simulink model "UR5"  (R2021a)
settings: Solver=ode45  StartTime=0.0  StopTime=duration  MaxStep=0.0001  RelTol=1e-3
values from neighbouring files (symbols this model uses):
  bound = 1e-6    (= 1e-06)    [parameter_setting.m]
  degree = 0.5    [parameter_setting.m]
  N = 2    [ICL_offline.m]
  rp = [-0.1 0 0.1]    [parameter_setting.m]
undefined symbols (not defined in the file or in its folder): DiscIntNeverNeededParam, Levenberg, Marquardt, sigbuilder_block, X, Y, Z
libraries: sm_lib x166, nesl_utility x41, robotmaniplib x2, SignalEditorBlockLib x2
(part 5 of 5)

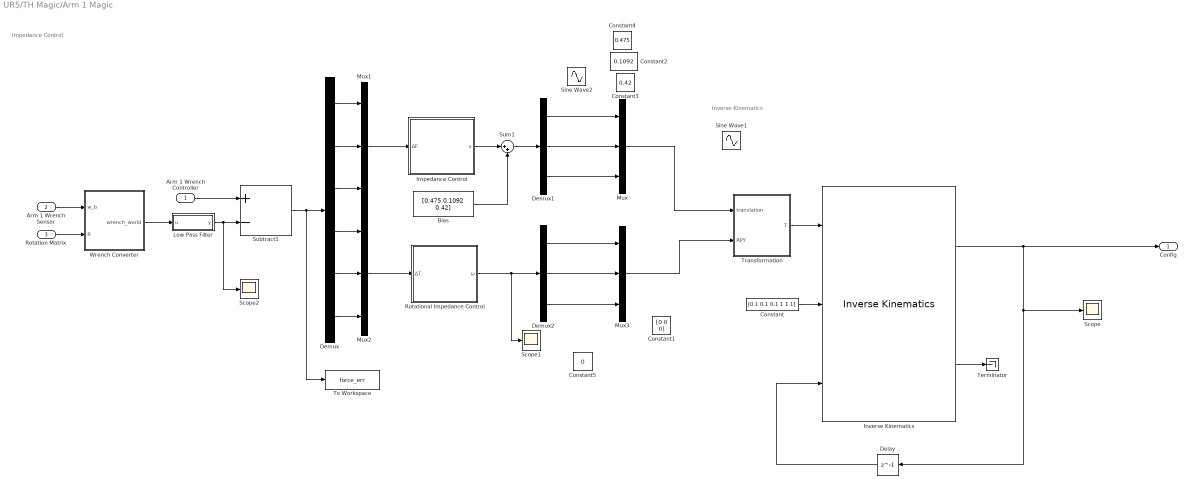
== system UR5/TH Magic/Arm 1 Magic ==
  note: Impedance Control
  note: Inverse Kinematics
  Arm 1 Wrench Controller : Inport
  Arm 1 Wrench Sensor : Inport  Port=2
  Rotation Matrix : Inport  Port=3
  Bias : Constant  Value=[0.475 0.1092 0.42]
  Constant : Constant  Value=[0.1 0.1 0.1 1 1 1]
  Constant1 : Constant  Value=[0 0 0]
  Constant2 : Constant  Value=0.1092
  Constant3 : Constant  Value=0.42
  Constant4 : Constant  Value=0.475
  Constant5 : Constant  Value=0
  Delay : Delay  DelayLength=1
  Demux : Demux  Outputs=6
  Demux1 : Demux  Outputs=3
  Demux2 : Demux  Outputs=3
  Impedance Control : Subsystem
  Inverse Kinematics : robotmaniplib/Inverse Kinematics  RigidBodyTree=robot  EndEffector=ee_link  ShowInfo=on  SolverName=Levenberg-Marquardt  EnforceJointLimits=on  MaxIterations=1500  MaxTime=10  GradientTolerance=1e-7  SolutionTolerance=1e-6  StepTolerance=1e-14  ErrorChangeTolerance=1e-12  UseErrorDamping=on  DampingBias=0.0025  SimulateUsing=Interpreted execution
  Low Pass Filter : MATLAB Function  TreatAsAtomicUnit=on
  Mux{,1..3} (4 alike) : Mux  Inputs=3
  Rotational Impedance Control : Subsystem
  Scope : Scope
  Scope1 : Scope
  Scope2 : Scope
  Sine Wave1 : Sin  Amplitude=0.2  Bias=0.475  Frequency=1.6  SampleTime=0
  Sine Wave2 : Sin  Amplitude=-0.2  Bias=0.475  Frequency=1.6  SampleTime=0
  Subtract1 : Sum  Inputs=+-
  Sum1 : Sum  Inputs=|++
  Terminator : Terminator
  To Workspace : ToWorkspace  VariableName=force_err  SaveFormat=Timeseries  SampleTime=-1
  Transformation : MATLAB Function  TreatAsAtomicUnit=on
  Wrench Converter : MATLAB Function  TreatAsAtomicUnit=on
  Config : Outport
  wires:
  Demux/3 -> Mux1/3
  Mux/1 -> Transformation/1(translation)
  Inverse Kinematics/1 -> Config/1, Delay/1, Scope/1
  Transformation/1(T) -> Inverse Kinematics/1
  Demux/6 -> Mux2/3
  Demux/5 -> Mux2/2
  Bias/1 -> Sum1/2
  Inverse Kinematics/2 -> Terminator/1
  Constant/1 -> Inverse Kinematics/2
  Demux/2 -> Mux1/2
  Delay/1 -> Inverse Kinematics/3
  Demux/1 -> Mux1/1
  Mux2/1 -> Rotational Impedance Control/1(ΔT)
  Rotational Impedance Control/1(ω) -> Scope1/1, Demux2/1
  Demux/4 -> Mux2/1
  Mux1/1 -> Impedance Control/1(ΔF)
  Demux1/3 -> Mux/3
  Subtract1/1 -> To Workspace/1, Demux/1
  Arm 1 Wrench Controller/1 -> Subtract1/1
  Arm 1 Wrench Sensor/1 -> Wrench Converter/1(w_b)
  Rotation Matrix/1 -> Wrench Converter/2(R)
  Sum1/1 -> Demux1/1
  Demux1/2 -> Mux/2
  Demux2/2 -> Mux3/2
  Demux2/1 -> Mux3/1
  Demux2/3 -> Mux3/3
  Demux1/1 -> Mux/1
  Impedance Control/1(x) -> Sum1/1
  Mux3/1 -> Transformation/2(RPY)
  Wrench Converter/1(wrench_world) -> Low Pass Filter/1(u)
  Low Pass Filter/1(y) -> Scope2/1, Subtract1/2

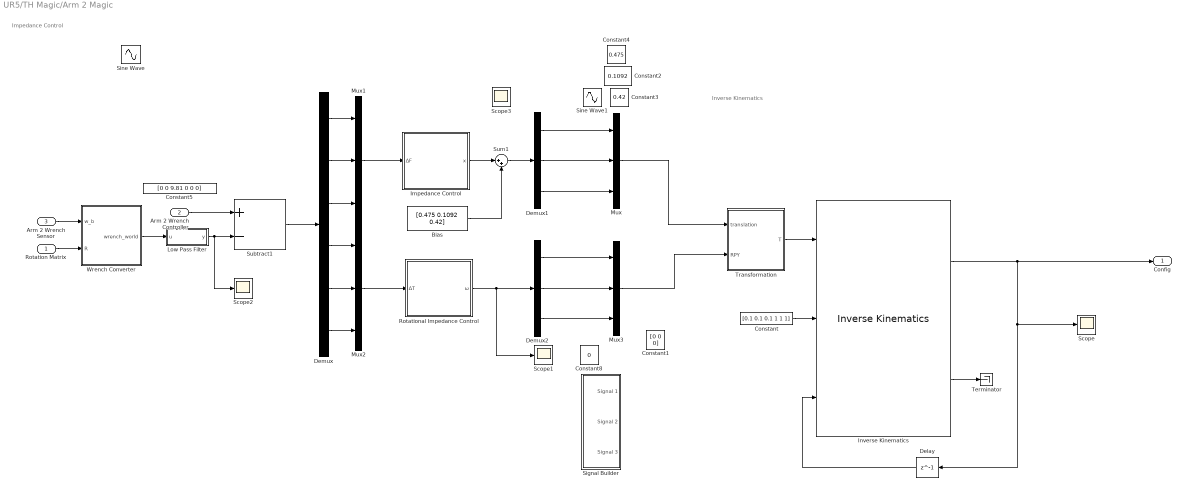
== system UR5/TH Magic/Arm 2 Magic ==
  note: Inverse Kinematics
  note: Impedance Control
  Rotation Matrix : Inport
  Arm 2 Wrench Controller : Inport  Port=2
  Arm 2 Wrench Sensor : Inport  Port=3
  Bias : Constant  Value=[0.475 0.1092 0.42]
  Constant : Constant  Value=[0.1 0.1 0.1 1 1 1]
  Constant1 : Constant  Value=[0 0 0]
  Constant2 : Constant  Value=0.1092
  Constant3 : Constant  Value=0.42
  Constant4 : Constant  Value=0.475
  Constant5 : Constant  Value=[0 0 9.81 0 0 0]
  Constant8 : Constant  Value=0
  Delay : Delay  DelayLength=1
  Demux : Demux  Outputs=6
  Demux1 : Demux  Outputs=3
  Demux2 : Demux  Outputs=3
  Impedance Control : Subsystem
  Inverse Kinematics : robotmaniplib/Inverse Kinematics  RigidBodyTree=robot  EndEffector=ee_link  ShowInfo=on  SolverName=Levenberg-Marquardt  EnforceJointLimits=on  MaxIterations=1500  MaxTime=10  GradientTolerance=1e-7  SolutionTolerance=1e-6  StepTolerance=1e-14  ErrorChangeTolerance=1e-12  UseErrorDamping=on  DampingBias=0.0025  SimulateUsing=Interpreted execution
  Low Pass Filter : MATLAB Function  TreatAsAtomicUnit=on
  Mux{,1..3} (4 alike) : Mux  Inputs=3
  Rotational Impedance Control : Subsystem
  Scope{,1..3} (4 alike) : Scope
  Signal Builder : Subsystem  Tag=STV Subsys  LoadFcn=sigbuilder_block('load');  StartFcn=sigbuilder_block('start');  StopFcn=sigbuilder_block('stop');  ClipboardFcn=sigbuilder_block('clipboard');  mask(Sigbuilder block){tuvar=[0:10]}
      mask help: Simulink:masks:SigbuilderBlock_MD
      mask init:
      | if ~strcmp(get_param(bdroot(gcbh),'SimulationStatus'),'stopped') tuvar = sigbuilder_block('maskInit'); end
      settings: CopyFcn=sigbuilder_block('copy');  DeleteFcn=sigbuilder_block('delete');  ModelCloseFcn=sigbuilder_block('modelClose');  PreSaveFcn=sigbuilder_block('preSave');  PauseFcn=sigbuilder_block('pause');  ContinueFcn=sigbuilder_block('continue');  NameChangeFcn=sigbuilder_block('namechange');  OpenFcn=sigbuilder_block('open',[437.6 199.2 550.4 400 ]);  CloseFcn=sigbuilder_block('close');
      mask Display: plot(0, 0, 100, 100,[2, 2, 32, 32, 2], [68, 8, 8, 68, 68],[32, 2], [38, 38], [32, 19, 2],[53, 60, 44], [32, 17, 17, 2],[16, 16, 31, 31]);txt = getActiveGroup(gcbh);text(2, 100, txt,'verticalAlignment', 'top');
  Sine Wave : Sin  Amplitude=0.1  SampleTime=0
  Sine Wave1 : Sin  Amplitude=-0.2  Bias=0.475  Frequency=1.6  SampleTime=0
  Subtract1 : Sum  Inputs=+-
  Sum1 : Sum  Inputs=|++
  Terminator : Terminator
  Transformation : MATLAB Function  TreatAsAtomicUnit=on
  Wrench Converter : MATLAB Function  TreatAsAtomicUnit=on
  Config : Outport
  wires:
  Demux/3 -> Mux1/3
  Mux/1 -> Transformation/1(translation)
  Inverse Kinematics/1 -> Scope/1, Delay/1, Config/1
  Transformation/1(T) -> Inverse Kinematics/1
  Demux/6 -> Mux2/3
  Demux/5 -> Mux2/2
  Bias/1 -> Sum1/2
  Inverse Kinematics/2 -> Terminator/1
  Constant/1 -> Inverse Kinematics/2
  Demux/2 -> Mux1/2
  Delay/1 -> Inverse Kinematics/3
  Demux/1 -> Mux1/1
  Mux2/1 -> Rotational Impedance Control/1(ΔT)
  Rotational Impedance Control/1(ω) -> Scope1/1, Demux2/1
  Demux/4 -> Mux2/1
  Mux1/1 -> Impedance Control/1(ΔF)
  Demux1/3 -> Mux/3
  Subtract1/1 -> Demux/1
  Demux1/1 -> Mux/1
  Rotation Matrix/1 -> Wrench Converter/2(R)
  Arm 2 Wrench Sensor/1 -> Wrench Converter/1(w_b)
  Arm 2 Wrench Controller/1 -> Subtract1/1
  Sum1/1 -> Demux1/1
  Demux1/2 -> Mux/2
  Demux2/1 -> Mux3/1
  Demux2/2 -> Mux3/2
  Demux2/3 -> Mux3/3
  Impedance Control/1(x) -> Sum1/1
  Mux3/1 -> Transformation/2(RPY)
  Wrench Converter/1(wrench_world) -> Low Pass Filter/1(u)
  Low Pass Filter/1(y) -> Scope2/1, Subtract1/2

== system UR5/Trajectory/Rotation ==
  Demux : Demux  Tag=STV Demux  Outputs=6
      settings: DisplayOption=none
  FromWs : FromWorkspace  Tag=STV FromWs  VariableName=tuvar
      SigBuilderData=|
      | common.afterFinalStr = 'Extrapolate'
      | common.sampleTime = 0
      | dataSet.timeRange = [0 10]
      | dataSet.name = 'Group 1'
      | sbobj.Groups.Name = 'Group 1'
      | sbobj.Groups.Signals(1).Name = 'wx'
      | sbobj.Groups.Signals(1).XData = [0 1 1 4 4 10]
      | sbobj.Groups.Signals(1).YData = [0 0 -0.4 -0.4 0 0]
      | sbobj.Groups.Signals(2).Name = 'wy'
      | sbobj.Groups.Signals(2).XData = [0 6 6 8 8 10]
      | sbobj.Groups.Signals(2).YData = [0 0 -0.2 -0.2 0 0]
      | sbobj.Groups.Signals(3).Name = 'wz'
      | sbobj.Groups.Signals(3).XData = [0 4 4 6 6 10]
      | sbobj.Groups.Signals(3).YData = [0 0 0.2 0.2 0 0]
      | sbobj.Groups.Signals(4).Name = 'alx'
      | sbobj.Groups.Signals(4).XData = [0 10]
      | sbobj.Groups.Signals(4).YData = [0 0]
      | sbobj.Groups.Signals(5).Name = 'aly'
      | sbobj.Groups.Signals(5).XData = [0 10]
      | sbobj.Groups.Signals(5).YData = [0 0]
      | sbobj.Groups.Signals(6).Name = 'alz'
      | sbobj.Groups.Signals(6).XData = [0 10]
      | sbobj.Groups.Signals(6).YData = [0 0]
  wx : Outport  Tag=STV Outport
  wy : Outport  Tag=STV Outport  Port=2
  wz : Outport  Tag=STV Outport  Port=3
  alx : Outport  Tag=STV Outport  Port=4
  aly : Outport  Tag=STV Outport  Port=5
  alz : Outport  Tag=STV Outport  Port=6
  wires:
  FromWs/1 -> Demux/1
  Demux/1 -> wx/1
  Demux/2 -> wy/1
  Demux/3 -> wz/1
  Demux/4 -> alx/1
  Demux/5 -> aly/1
  Demux/6 -> alz/1

== system UR5/Trajectory/Rotation1 ==
  Demux : Demux  Tag=STV Demux  Outputs=6
      settings: DisplayOption=none
  FromWs : FromWorkspace  Tag=STV FromWs  VariableName=tuvar
      SigBuilderData=|
      | common.afterFinalStr = 'Extrapolate'
      | common.sampleTime = 0
      | dataSet.timeRange = [0 10]
      | dataSet.name = 'Group 2'
      | sbobj.Groups.Name = 'Group 2'
      | sbobj.Groups.Signals(1).Name = 'wx'
      | sbobj.Groups.Signals(1).XData = [0 1 4 10]
      | sbobj.Groups.Signals(1).YData = [0 0 0 0]
      | sbobj.Groups.Signals(2).Name = 'wy'
      | sbobj.Groups.Signals(2).XData = [0 6 8 10]
      | sbobj.Groups.Signals(2).YData = [0 0 0 0]
      | sbobj.Groups.Signals(3).Name = 'wz'
      | sbobj.Groups.Signals(3).XData = [0 4 6 10]
      | sbobj.Groups.Signals(3).YData = [0 0 0 0]
      | sbobj.Groups.Signals(4).Name = 'alx'
      | sbobj.Groups.Signals(4).XData = [0 10]
      | sbobj.Groups.Signals(4).YData = [0 0]
      | sbobj.Groups.Signals(5).Name = 'aly'
      | sbobj.Groups.Signals(5).XData = [0 10]
      | sbobj.Groups.Signals(5).YData = [0 0]
      | sbobj.Groups.Signals(6).Name = 'alz'
      | sbobj.Groups.Signals(6).XData = [0 10]
      | sbobj.Groups.Signals(6).YData = [0 0]
  wx : Outport  Tag=STV Outport
  wy : Outport  Tag=STV Outport  Port=2
  wz : Outport  Tag=STV Outport  Port=3
  alx : Outport  Tag=STV Outport  Port=4
  aly : Outport  Tag=STV Outport  Port=5
  alz : Outport  Tag=STV Outport  Port=6
  wires:
  FromWs/1 -> Demux/1
  Demux/1 -> wx/1
  Demux/2 -> wy/1
  Demux/3 -> wz/1
  Demux/4 -> alx/1
  Demux/5 -> aly/1
  Demux/6 -> alz/1

== system UR5/Trajectory/Rotation2 ==
  Demux : Demux  Tag=STV Demux  Outputs=6
      settings: DisplayOption=none
  FromWs : FromWorkspace  Tag=STV FromWs  VariableName=tuvar
      SigBuilderData=|
      | common.afterFinalStr = 'Extrapolate'
      | common.sampleTime = 0
      | dataSet.timeRange = [0 100]
      | dataSet.name = 'Group 3'
      | sbobj.Groups.Name = 'Group 3'
      | sbobj.Groups.Signals(1).Name = 'wx'
      | sbobj.Groups.Signals(1).XData = [0 2.5 2.5 5 5 7.5 7.5 10 10 12.5 12.5 15 15 17.5 17.5 20 20 22.5 22.5 25 25 27.5 27.5 30 30 32.5 32.5 35 35 37.5 37.5 40 40 42.5 42.5 45 45 47.5 47.5 50 50 52.5 52.5 55 55 57.5 57.5 60 60 62.5 62.5 65 65 67.5 67.5 70 70 72.5 72.5 75 75 77.5 77.5 80 80 82.5 82.5 85 85 87.5 87.5 90 90 92.5 92.5 95 95 97.5 97.5 100]
      | sbobj.Groups.Signals(1).YData = [0.4 0.4 -0.4 -0.4 0.4 0.4 -0.4 -0.4 0.4 0.4 -0.4 -0.4 0.4 0.4 -0.4 -0.4 0.4 0.4 -0.4 -0.4 0.4 0.4 -0.4 -0.4 0.4 0.4 -0.4 -0.4 0.4 0.4 -0.4 -0.4 0.4 0.4 -0.4 -0.4 0.4 0.4 -0.4 -0.4 0.4 0.4 -0.4 -0.4 0.4 0.4 -0.4 -0.4 0.4 0.4 -0.4 -0.4 0.4 0.4 -0.4 -0.4 0.4 0.4 -0.4 -0.4 0.4 0.4 -0.4 -0.4 0.4 0.4 -0.4 -0.4 0.4 0.4 -0.4 -0.4 0.4 0.4 -0.4 -0.4 0.4 0.4 -0.4 -0.4]
      | sbobj.Groups.Signals(2).Name = 'wy'
      | sbobj.Groups.Signals(2).XData = [0 1.5 1.5 3.5 3.5 5.5 5.5 7.5 7.5 9.5 9.5 11.5 11.5 13.5 13.5 15.5 15.5 17.5 17.5 19.5 19.5 21.5 21.5 23.5 23.5 25.5 25.5 27.5 27.5 29.5 29.5 31.5 31.5 33.5 33.5 35.5 35.5 37.5 37.5 39.5 39.5 41.5 41.5 43.5 43.5 45.5 45.5 47.5 47.5 49.5 49.5 51.5 51.5 53.5 53.5 55.5 55.5 57.5 57.5 59.5 59.5 61.5 61.5 63.5 63.5 65.5 65.5 67.5 67.5 69.5 69.5 71.5 71.5 73.5 73.5 75.5 75.5 77.5 77.5 79.5 79.5 81.5 81.5 83.5 83.5 85.5 85.5 87.5 87.5 89.5 89.5 91.5 91.5 93.5 93.5 95.5 95.5 97.5 97.5 100]
      | sbobj.Groups.Signals(2).YData = [0.1 0.1 -0.1 -0.1 0.1 0.1 -0.1 -0.1 0.1 0.1 -0.1 -0.1 0.1 0.1 -0.1 -0.1 0.1 0.1 -0.1 -0.1 0.1 0.1 -0.1 -0.1 0.1 0.1 -0.1 -0.1 0.1 0.1 -0.1 -0.1 0.1 0.1 -0.1 -0.1 0.1 0.1 -0.1 -0.1 0.1 0.1 -0.1 -0.1 0.1 0.1 -0.1 -0.1 0.1 0.1 -0.1 -0.1 0.1 0.1 -0.1 -0.1 0.1 0.1 -0.1 -0.1 0.1 0.1 -0.1 -0.1 0.1 0.1 -0.1 -0.1 0.1 0.1 -0.1 -0.1 0.1 0.1 -0.1 -0.1 0.1 0.1 -0.1 -0.1 0.1 0.1 -0.1 -0.1 0.1 0.1 -0.1 -0.1 0.1 0.1 -0.1 -0.1 0.1 0.1 -0.1 -0.1 0.1 0.1 -0.1 -0.1]
      | sbobj.Groups.Signals(3).Name = 'wz'
      | sbobj.Groups.Signals(3).XData = [0 5 5 10 10 15 15 20 20 25 25 30 30 35 35 40 40 45 45 50 50 55 55 60 60 65 65 70 70 75 75 80 80 85 85 90 90 95 95 100]
      | sbobj.Groups.Signals(3).YData = [0.05 0.05 -0.05 -0.05 0.05 0.05 -0.05 -0.05 0.15 0.15 -0.15 -0.15 0.15 0.15 -0.15 -0.15 0.15 0.15 -0.15 -0.15 0.15 0.15 -0.15 -0.15 0.15 0.15 -0.15 -0.15 0.15 0.15 -0.15 -0.15 0.15 0.15 -0.15 -0.15 0.15 0.15 -0.15 -0.15]
      | sbobj.Groups.Signals(4).Name = 'alx'
      | sbobj.Groups.Signals(4).XData = [0 100]
      | sbobj.Groups.Signals(4).YData = [0 0]
      | sbobj.Groups.Signals(5).Name = 'aly'
      | sbobj.Groups.Signals(5).XData = [0 100]
      | sbobj.Groups.Signals(5).YData = [0 0]
      | sbobj.Groups.Signals(6).Name = 'alz'
      | sbobj.Groups.Signals(6).XData = [0 100]
      | sbobj.Groups.Signals(6).YData = [0 0]
      | sbobj.Groups.TimeRange = [0 100]
  wx : Outport  Tag=STV Outport
  wy : Outport  Tag=STV Outport  Port=2
  wz : Outport  Tag=STV Outport  Port=3
  alx : Outport  Tag=STV Outport  Port=4
  aly : Outport  Tag=STV Outport  Port=5
  alz : Outport  Tag=STV Outport  Port=6
  wires:
  FromWs/1 -> Demux/1
  Demux/1 -> wx/1
  Demux/2 -> wy/1
  Demux/3 -> wz/1
  Demux/4 -> alx/1
  Demux/5 -> aly/1
  Demux/6 -> alz/1

== system UR5/Trajectory/Translation ==
  Demux : Demux  Tag=STV Demux  Outputs=6
      settings: DisplayOption=none
  FromWs : FromWorkspace  Tag=STV FromWs  VariableName=tuvar
      SigBuilderData=|
      | common.afterFinalStr = 'Extrapolate'
      | common.sampleTime = 0
      | dataSet.timeRange = [0 10]
      | dataSet.name = 'Group 1'
      | sbobj.Groups.Name = 'Group 1'
      | sbobj.Groups.Signals(1).Name = 'vx'
      | sbobj.Groups.Signals(1).XData = [0 1.2 1.2 2 2 10]
      | sbobj.Groups.Signals(1).YData = [0.3 0.3 -0.3 -0.3 0 0]
      | sbobj.Groups.Signals(2).Name = 'vy'
      | sbobj.Groups.Signals(2).XData = [0 2 4 6 8 10]
      | sbobj.Groups.Signals(2).YData = [-0.5 0.5 -0.5 0.5 -0.5 0.5]
      | sbobj.Groups.Signals(3).Name = 'vz'
      | sbobj.Groups.Signals(3).XData = [0 3.01 3.01 4 4 5.01 5.01 10]
      | sbobj.Groups.Signals(3).YData = [0 0 0.3 0.3 -0.3 -0.3 0 0]
      | sbobj.Groups.Signals(4).Name = 'ax'
      | sbobj.Groups.Signals(4).XData = [0 10]
      | sbobj.Groups.Signals(4).YData = [0 0]
      | sbobj.Groups.Signals(5).Name = 'ay'
      | sbobj.Groups.Signals(5).XData = [0 2 2 4 4 6 6 8 8 10]
      | sbobj.Groups.Signals(5).YData = [0.5 0.5 -0.5 -0.5 0.5 0.5 -0.5 -0.5 0.5 0.5]
      | sbobj.Groups.Signals(6).Name = 'az'
      | sbobj.Groups.Signals(6).XData = [0 10]
      | sbobj.Groups.Signals(6).YData = [0 0]
  vx : Outport  Tag=STV Outport
  vy : Outport  Tag=STV Outport  Port=2
  vz : Outport  Tag=STV Outport  Port=3
  ax : Outport  Tag=STV Outport  Port=4
  ay : Outport  Tag=STV Outport  Port=5
  az : Outport  Tag=STV Outport  Port=6
  wires:
  Demux/1 -> vx/1
  FromWs/1 -> Demux/1
  Demux/2 -> vy/1
  Demux/3 -> vz/1
  Demux/4 -> ax/1
  Demux/5 -> ay/1
  Demux/6 -> az/1

== system UR5/Trajectory/Translation1 ==
  Demux : Demux  Tag=STV Demux  Outputs=6
      settings: DisplayOption=none
  FromWs : FromWorkspace  Tag=STV FromWs  VariableName=tuvar
      SigBuilderData=|
      | common.afterFinalStr = 'Extrapolate'
      | common.sampleTime = 0
      | dataSet.timeRange = [0 10]
      | dataSet.name = 'Group 2'
      | sbobj.Groups.Name = 'Group 2'
      | sbobj.Groups.Signals(1).Name = 'vx'
      | sbobj.Groups.Signals(1).XData = [0 10]
      | sbobj.Groups.Signals(1).YData = [0 0]
      | sbobj.Groups.Signals(2).Name = 'vy'
      | sbobj.Groups.Signals(2).XData = [0 10]
      | sbobj.Groups.Signals(2).YData = [0 0]
      | sbobj.Groups.Signals(3).Name = 'vz'
      | sbobj.Groups.Signals(3).XData = [0 10]
      | sbobj.Groups.Signals(3).YData = [0 0]
      | sbobj.Groups.Signals(4).Name = 'ax'
      | sbobj.Groups.Signals(4).XData = [0 10]
      | sbobj.Groups.Signals(4).YData = [0 0]
      | sbobj.Groups.Signals(5).Name = 'ay'
      | sbobj.Groups.Signals(5).XData = [0 10]
      | sbobj.Groups.Signals(5).YData = [0 0]
      | sbobj.Groups.Signals(6).Name = 'az'
      | sbobj.Groups.Signals(6).XData = [0 10]
      | sbobj.Groups.Signals(6).YData = [0 0]
  vx : Outport  Tag=STV Outport
  vy : Outport  Tag=STV Outport  Port=2
  vz : Outport  Tag=STV Outport  Port=3
  ax : Outport  Tag=STV Outport  Port=4
  ay : Outport  Tag=STV Outport  Port=5
  az : Outport  Tag=STV Outport  Port=6
  wires:
  Demux/1 -> vx/1
  FromWs/1 -> Demux/1
  Demux/2 -> vy/1
  Demux/3 -> vz/1
  Demux/4 -> ax/1
  Demux/5 -> ay/1
  Demux/6 -> az/1

== system UR5/Trajectory/Translation2 ==
  Demux : Demux  Tag=STV Demux  Outputs=8
      settings: DisplayOption=none
  FromWs : FromWorkspace  Tag=STV FromWs  VariableName=tuvar
      SigBuilderData=|
      | common.afterFinalStr = 'Extrapolate'
      | common.sampleTime = 0
      | dataSet.timeRange = [0 100]
      | dataSet.name = 'Group 3'
      | sbobj.Groups.Name = 'Group 3'
      | sbobj.Groups.Signals(1).Name = 'vx'
      | sbobj.Groups.Signals(1).XData = [0 1.25 1.25 2.5 2.5 3.75 3.75 5 5 6.25 6.25 7.5 7.5 8.75 8.75 10 10 11.25 11.25 12.5 12.5 13.75 13.75 15 15 16.25 16.25 17.5 17.5 18.75 18.75 20 20 21.25 21.25 22.5 22.5 23.75 23.75 25 25 26.25 26.25 27.5 27.5 28.75 28.75 30 30 31.25 31.25 32.5 32.5 33.75 33.75 35 35 36.25 36.25 37.5 37.5 38.75 38.75 40 40 41.25 41.25 42.5 42.5 43.75 43.75 45 45 46.25 46.25 47.5 47.5 48.75 48.75 50 50 51.25 51.25 52.5 52.5 53.75 53.75 55 55 56.25 56.25 57.5 57.5 58.75 58.75 60 60 61.25 61.25 62.5 62.5 63.75 63.75 65 65 66.25 66.25 67.5 67.5 68.75 68.75 70 70 71.25 71.25 72.5 72.5 73.75 73.75 75 75 76.25 76.25 77.5 77.5 78.75 78.75 80 80 81.25 81.25 82.5 82.5 83.75 83.75 85 85 86.25 86.25 87.5 87.5 88.75 88.75 90 90 91.25 91.25 92.5 92.5 93.75 93.75 95 95 96.25 96.25 97.5 97.5 98.75 98.75 100]
      | sbobj.Groups.Signals(1).YData = [0.1 0.1 -0.1 -0.1 0.1 0.1 -0.1 -0.1 0.1 0.1 -0.1 -0.1 0.1 0.1 -0.1 -0.1 0.1 0.1 -0.1 -0.1 0.1 0.1 -0.1 -0.1 0.1 0.1 -0.1 -0.1 0.1 0.1 -0.1 -0.1 0.1 0.1 -0.1 -0.1 0.1 0.1 -0.1 -0.1 0.1 0.1 -0.1 -0.1 0.1 0.1 -0.1 -0.1 0.1 0.1 -0.1 -0.1 0.1 0.1 -0.1 -0.1 0.1 0.1 -0.1 -0.1 0.1 0.1 -0.1 -0.1 0.1 0.1 -0.1 -0.1 0.1 0.1 -0.1 -0.1 0.1 0.1 -0.1 -0.1 0.1 0.1 -0.1 -0.1 0.1 0.1 -0.1 -0.1 0.1 0.1 -0.1 -0.1 0.1 0.1 -0.1 -0.1 0.1 0.1 -0.1 -0.1 0.1 0.1 -0.1 -0.1 0.1 0.1 -0.1 -0.1 0.1 0.1 -0.1 -0.1 0.1 0.1 -0.1 -0.1 0.1 0.1 -0.1 -0.1 0.1 0.1 -0.1 -0.1 0.1 0.1 -0.1 -0.1 0.1 0.1 -0.1 -0.1 0.1 0.1 -0.1 -0.1 0.1 0.1 -0.1 -0.1 0.1 0.1 -0.1 -0.1 0.1 0.1 -0.1 -0.1 0.1 0.1 -0.1 -0.1 0.1 0.1 -0.1 -0.1 0.1 0.1 -0.1 -0.1 0.1 0.1 -0.1 -0.1]
      | sbobj.Groups.Signals(2).Name = 'vy'
      | sbobj.Groups.Signals(2).XData = [0 100]
      | sbobj.Groups.Signals(2).YData = [0 0]
      | sbobj.Groups.Signals(3).Name = 'vz'
      | sbobj.Groups.Signals(3).XData = [0 5 5 10 10 15 15 20 20 25 25 30 30 35 35 40 40 45 45 50 50 55 55 60 60 65 65 70 70 75 75 80 80 85 85 90 90 95 95 100]
      | sbobj.Groups.Signals(3).YData = [0 0 -0.05 -0.05 0.05 0.05 -0.05 -0.05 0.05 0.05 -0.05 -0.05 0.05 0.05 -0.05 -0.05 0.05 0.05 -0.05 -0.05 0.05 0.05 -0.05 -0.05 0.05 0.05 -0.05 -0.05 0.05 0.05 -0.05 -0.05 0.05 0.05 -0.05 -0.05 0.05 0.05 -0.05 -0.05]
      | sbobj.Groups.Signals(4).Name = 'ax'
      | sbobj.Groups.Signals(4).XData = [0 100]
      | sbobj.Groups.Signals(4).YData = [0 0]
      | sbobj.Groups.Signals(5).Name = 'ay'
      | sbobj.Groups.Signals(5).XData = [0 100]
      | sbobj.Groups.Signals(5).YData = [0 0]
      | sbobj.Groups.Signals(6).Name = 'az'
      | sbobj.Groups.Signals(6).XData = [0 100]
      | sbobj.Groups.Signals(6).YData = [0 0]
      | sbobj.Groups.Signals(7).Name = 'vy1'
      | sbobj.Groups.Signals(7).XData = [0 2 4 6 8 10 12 14 16 18 20 22 24 26 28 30 32 34 36 38 40 42 44 46 48 50 52 54 56 58 60 62 64 66 68 70 72 74 76 78 80 82 84 86 88 90 92 94 96 98 100]
      | sbobj.Groups.Signals(7).YData = [-0.5 0.5 -0.5 0.5 -0.5 0.5 -0.5 0.5 -0.5 0.5 -0.5 0.5 -0.5 0.5 -0.5 0.5 -0.5 0.5 -0.5 0.5 -0.5 0.5 -0.5 0.5 -0.5 0.5 -0.5 0.5 -0.5 0.5 -0.5 0.5 -0.5 0.5 -0.5 0.5 -0.5 0.5 -0.5 0.5 -0.5 0.5 -0.5 0.5 -0.5 0.5 -0.5 0.5 -0.5 0.5 -0.5]
      | sbobj.Groups.Signals(8).Name = 'ay1'
      | sbobj.Groups.Signals(8).XData = [0 2 2 4 4 6 6 8 8 10 10 12 12 14 14 16 16 18 18 20 20 22 22 24 24 26 26 28 28 30 30 32 32 34 34 36 36 38 38 40 40 42 42 44 44 46 46 48 48 50 50 52 52 54 54 56 56 58 58 60 60 62 62 64 64 66 66 68 68 70 70 72 72 74 74 76 76 78 78 80 80 82 82 84 84 86 86 88 88 90 90 92 92 94 94 96 96 98 98 100]
      | sbobj.Groups.Signals(8).YData = [0.5 0.5 -0.5 -0.5 0.5 0.5 -0.5 -0.5 0.5 0.5 -0.5 -0.5 0.5 0.5 -0.5 -0.5 0.5 0.5 -0.5 -0.5 0.5 0.5 -0.5 -0.5 0.5 0.5 -0.5 -0.5 0.5 0.5 -0.5 -0.5 0.5 0.5 -0.5 -0.5 0.5 0.5 -0.5 -0.5 0.5 0.5 -0.5 -0.5 0.5 0.5 -0.5 -0.5 0.5 0.5 -0.5 -0.5 0.5 0.5 -0.5 -0.5 0.5 0.5 -0.5 -0.5 0.5 0.5 -0.5 -0.5 0.5 0.5 -0.5 -0.5 0.5 0.5 -0.5 -0.5 0.5 0.5 -0.5 -0.5 0.5 0.5 -0.5 -0.5 0.5 0.5 -0.5 -0.5 0.5 0.5 -0.5 -0.5 0.5 0.5 -0.5 -0.5 0.5 0.5 -0.5 -0.5 0.5 0.5 -0.5 -0.5]
      | sbobj.Groups.TimeRange = [0 100]
  vx : Outport  Tag=STV Outport
  vy : Outport  Tag=STV Outport  Port=2
  vz : Outport  Tag=STV Outport  Port=3
  ax : Outport  Tag=STV Outport  Port=4
  ay : Outport  Tag=STV Outport  Port=5
  az : Outport  Tag=STV Outport  Port=6
  vy1 : Outport  Tag=STV Outport  Port=7
  ay1 : Outport  Tag=STV Outport  Port=8
  wires:
  Demux/1 -> vx/1
  FromWs/1 -> Demux/1
  Demux/2 -> vy/1
  Demux/3 -> vz/1
  Demux/4 -> ax/1
  Demux/5 -> ay/1
  Demux/6 -> az/1
  Demux/7 -> vy1/1
  Demux/8 -> ay1/1

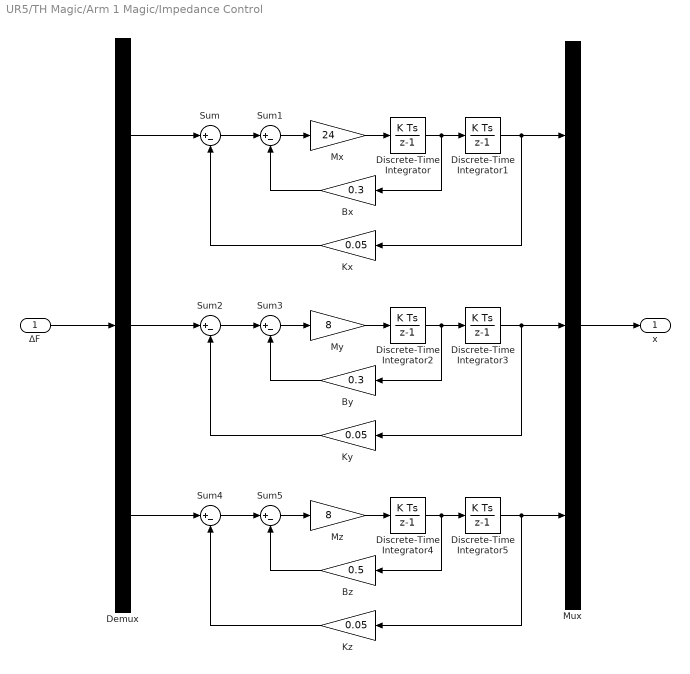
== system UR5/TH Magic/Arm 1 Magic/Impedance Control ==
  ΔF : Inport
  Bx : Gain  Gain=0.3
  By : Gain  Gain=0.3
  Bz : Gain  Gain=0.5
  Demux : Demux  Outputs=3
  Discrete-Time Integrator{,1..5} (6 alike) : DiscreteIntegrator  SampleTime=-1  ICPrevOutput=DiscIntNeverNeededParam  ICPrevScaledInput=DiscIntNeverNeededParam
  Kx : Gain  Gain=0.05
  Ky : Gain  Gain=0.05
  Kz : Gain  Gain=0.05
  Mux : Mux  Inputs=3
  Mx : Gain  Gain=24
  My : Gain  Gain=8
  Mz : Gain  Gain=8
  Sum{,1..5} (6 alike) : Sum  Inputs=|+-
  x : Outport
  wires:
  Bx/1 -> Sum1/2
  Mx/1 -> Discrete-Time Integrator/1
  Discrete-Time Integrator/1 -> Bx/1, Discrete-Time Integrator1/1
  Sum/1 -> Sum1/1
  Kx/1 -> Sum/2
  Sum1/1 -> Mx/1
  Discrete-Time Integrator1/1 -> Mux/1, Kx/1
  Discrete-Time Integrator3/1 -> Mux/2, Ky/1
  Ky/1 -> Sum2/2
  Sum2/1 -> Sum3/1
  Sum3/1 -> My/1
  Discrete-Time Integrator2/1 -> By/1, Discrete-Time Integrator3/1
  My/1 -> Discrete-Time Integrator2/1
  By/1 -> Sum3/2
  Discrete-Time Integrator5/1 -> Mux/3, Kz/1
  Kz/1 -> Sum4/2
  Sum4/1 -> Sum5/1
  Sum5/1 -> Mz/1
  Discrete-Time Integrator4/1 -> Bz/1, Discrete-Time Integrator5/1
  Mz/1 -> Discrete-Time Integrator4/1
  Bz/1 -> Sum5/2
  ΔF/1 -> Demux/1
  Demux/1 -> Sum/1
  Demux/2 -> Sum2/1
  Demux/3 -> Sum4/1
  Mux/1 -> x/1

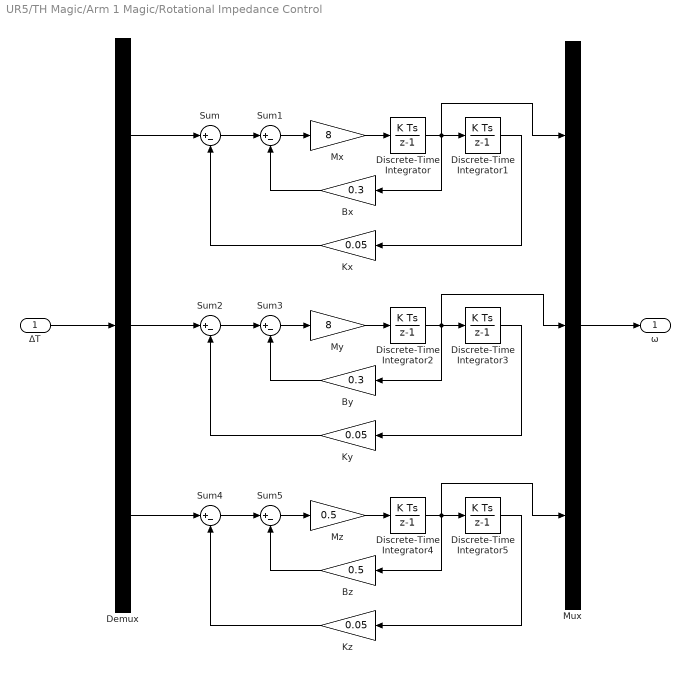
== system UR5/TH Magic/Arm 1 Magic/Rotational Impedance Control ==
  ΔT : Inport
  Bx : Gain  Gain=0.3
  By : Gain  Gain=0.3
  Bz : Gain  Gain=0.5
  Demux : Demux  Outputs=3
  Discrete-Time Integrator{,1..5} (6 alike) : DiscreteIntegrator  SampleTime=-1  ICPrevOutput=DiscIntNeverNeededParam  ICPrevScaledInput=DiscIntNeverNeededParam
  Kx : Gain  Gain=0.05
  Ky : Gain  Gain=0.05
  Kz : Gain  Gain=0.05
  Mux : Mux  Inputs=3
  Mx : Gain  Gain=8
  My : Gain  Gain=8
  Mz : Gain  Gain=0.5
  Sum{,1..5} (6 alike) : Sum  Inputs=|+-
  ω : Outport
  wires:
  Bx/1 -> Sum1/2
  Mx/1 -> Discrete-Time Integrator/1
  Discrete-Time Integrator/1 -> Mux/1, Bx/1, Discrete-Time Integrator1/1
  Sum/1 -> Sum1/1
  Kx/1 -> Sum/2
  Sum1/1 -> Mx/1
  Discrete-Time Integrator1/1 -> Kx/1
  Discrete-Time Integrator3/1 -> Ky/1
  Ky/1 -> Sum2/2
  Sum2/1 -> Sum3/1
  Sum3/1 -> My/1
  Discrete-Time Integrator2/1 -> By/1, Mux/2, Discrete-Time Integrator3/1
  My/1 -> Discrete-Time Integrator2/1
  By/1 -> Sum3/2
  Discrete-Time Integrator5/1 -> Kz/1
  Kz/1 -> Sum4/2
  Sum4/1 -> Sum5/1
  Sum5/1 -> Mz/1
  Discrete-Time Integrator4/1 -> Bz/1, Mux/3, Discrete-Time Integrator5/1
  Mz/1 -> Discrete-Time Integrator4/1
  Bz/1 -> Sum5/2
  ΔT/1 -> Demux/1
  Demux/1 -> Sum/1
  Demux/2 -> Sum2/1
  Demux/3 -> Sum4/1
  Mux/1 -> ω/1

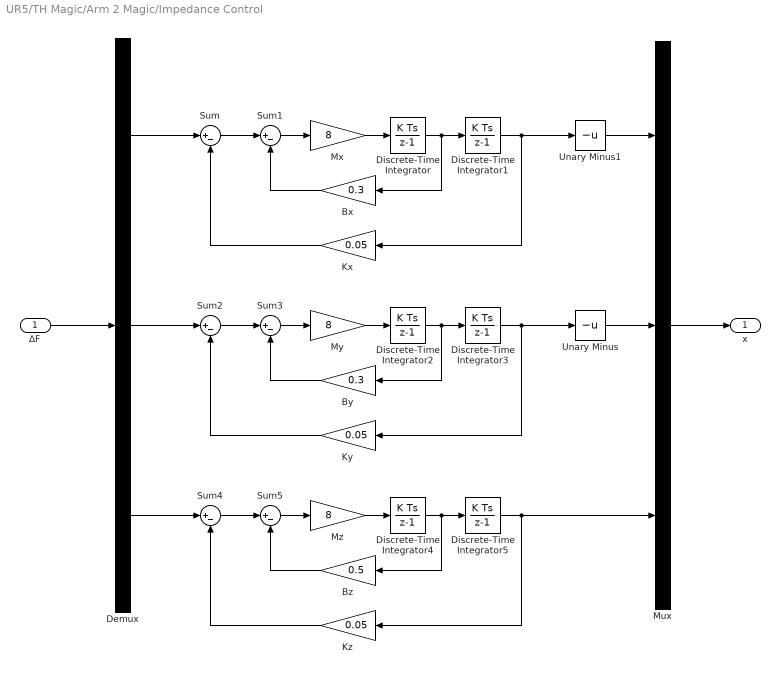
== system UR5/TH Magic/Arm 2 Magic/Impedance Control ==
  ΔF : Inport
  Bx : Gain  Gain=0.3
  By : Gain  Gain=0.3
  Bz : Gain  Gain=0.5
  Demux : Demux  Outputs=3
  Discrete-Time Integrator{,1..5} (6 alike) : DiscreteIntegrator  SampleTime=-1  ICPrevOutput=DiscIntNeverNeededParam  ICPrevScaledInput=DiscIntNeverNeededParam
  Kx : Gain  Gain=0.05
  Ky : Gain  Gain=0.05
  Kz : Gain  Gain=0.05
  Mux : Mux  Inputs=3
  Mx : Gain  Gain=8
  My : Gain  Gain=8
  Mz : Gain  Gain=8
  Sum{,1..5} (6 alike) : Sum  Inputs=|+-
  Unary Minus : UnaryMinus
  Unary Minus1 : UnaryMinus
  x : Outport
  wires:
  Bx/1 -> Sum1/2
  Mx/1 -> Discrete-Time Integrator/1
  Discrete-Time Integrator/1 -> Bx/1, Discrete-Time Integrator1/1
  Sum/1 -> Sum1/1
  Kx/1 -> Sum/2
  Sum1/1 -> Mx/1
  Discrete-Time Integrator1/1 -> Kx/1, Unary Minus1/1
  Discrete-Time Integrator3/1 -> Ky/1, Unary Minus/1
  Ky/1 -> Sum2/2
  Sum2/1 -> Sum3/1
  Sum3/1 -> My/1
  Discrete-Time Integrator2/1 -> By/1, Discrete-Time Integrator3/1
  My/1 -> Discrete-Time Integrator2/1
  By/1 -> Sum3/2
  Discrete-Time Integrator5/1 -> Kz/1, Mux/3
  Kz/1 -> Sum4/2
  Sum4/1 -> Sum5/1
  Sum5/1 -> Mz/1
  Discrete-Time Integrator4/1 -> Bz/1, Discrete-Time Integrator5/1
  Mz/1 -> Discrete-Time Integrator4/1
  Bz/1 -> Sum5/2
  ΔF/1 -> Demux/1
  Demux/1 -> Sum/1
  Demux/2 -> Sum2/1
  Demux/3 -> Sum4/1
  Mux/1 -> x/1
  Unary Minus/1 -> Mux/2
  Unary Minus1/1 -> Mux/1

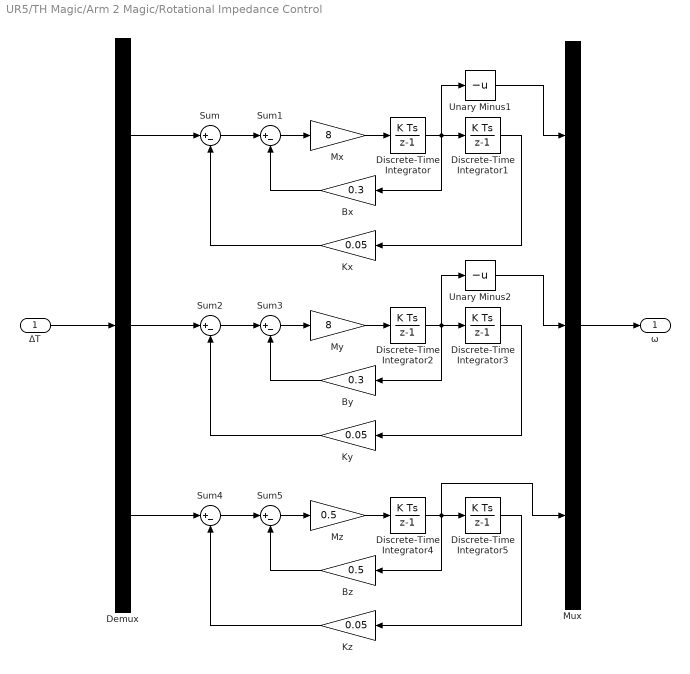
== system UR5/TH Magic/Arm 2 Magic/Rotational Impedance Control ==
  ΔT : Inport
  Bx : Gain  Gain=0.3
  By : Gain  Gain=0.3
  Bz : Gain  Gain=0.5
  Demux : Demux  Outputs=3
  Discrete-Time Integrator{,1..5} (6 alike) : DiscreteIntegrator  SampleTime=-1  ICPrevOutput=DiscIntNeverNeededParam  ICPrevScaledInput=DiscIntNeverNeededParam
  Kx : Gain  Gain=0.05
  Ky : Gain  Gain=0.05
  Kz : Gain  Gain=0.05
  Mux : Mux  Inputs=3
  Mx : Gain  Gain=8
  My : Gain  Gain=8
  Mz : Gain  Gain=0.5
  Sum{,1..5} (6 alike) : Sum  Inputs=|+-
  Unary Minus1 : UnaryMinus
  Unary Minus2 : UnaryMinus
  ω : Outport
  wires:
  Bx/1 -> Sum1/2
  Mx/1 -> Discrete-Time Integrator/1
  Sum/1 -> Sum1/1
  Kx/1 -> Sum/2
  Sum1/1 -> Mx/1
  Discrete-Time Integrator1/1 -> Kx/1
  Discrete-Time Integrator3/1 -> Ky/1
  Ky/1 -> Sum2/2
  Sum2/1 -> Sum3/1
  Sum3/1 -> My/1
  Discrete-Time Integrator2/1 -> By/1, Unary Minus2/1, Discrete-Time Integrator3/1
  My/1 -> Discrete-Time Integrator2/1
  By/1 -> Sum3/2
  Discrete-Time Integrator5/1 -> Kz/1
  Kz/1 -> Sum4/2
  Sum4/1 -> Sum5/1
  Sum5/1 -> Mz/1
  Discrete-Time Integrator4/1 -> Bz/1, Mux/3, Discrete-Time Integrator5/1
  Mz/1 -> Discrete-Time Integrator4/1
  Bz/1 -> Sum5/2
  ΔT/1 -> Demux/1
  Demux/1 -> Sum/1
  Demux/2 -> Sum2/1
  Demux/3 -> Sum4/1
  Mux/1 -> ω/1
  Unary Minus2/1 -> Mux/2
  Discrete-Time Integrator/1 -> Unary Minus1/1, Bx/1, Discrete-Time Integrator1/1
  Unary Minus1/1 -> Mux/1

== system UR5/TH Magic/Arm 2 Magic/Signal Builder ==
  Demux : Demux  Tag=STV Demux  Outputs=3
      settings: DisplayOption=none
  FromWs : FromWorkspace  Tag=STV FromWs  VariableName=tuvar
      SigBuilderData=|
      | common.afterFinalStr = 'Extrapolate'
      | common.sampleTime = 0
      | dataSet.timeRange = [0 10]
      | dataSet.name = 'Group 1'
      | sbobj.Groups.Name = 'Group 1'
      | sbobj.Groups.Signals(1).Name = 'Signal 1'
      | sbobj.Groups.Signals(1).XData = [0 1 3.8 4.5 10]
      | sbobj.Groups.Signals(1).YData = [0 0 0.02 0 0]
      | sbobj.Groups.Signals(2).Name = 'Signal 2'
      | sbobj.Groups.Signals(2).XData = [0 10]
      | sbobj.Groups.Signals(2).YData = [0 0]
      | sbobj.Groups.Signals(3).Name = 'Signal 3'
      | sbobj.Groups.Signals(3).XData = [0 10]
      | sbobj.Groups.Signals(3).YData = [0 0]
  Signal 1 : Outport  Tag=STV Outport
  Signal 2 : Outport  Tag=STV Outport  Port=2
  Signal 3 : Outport  Tag=STV Outport  Port=3
  wires:
  Demux/1 -> Signal 1/1
  FromWs/1 -> Demux/1
  Demux/2 -> Signal 2/1
  Demux/3 -> Signal 3/1

== matlab function UR5/Low pass filter ==
  settings: updateMethod=DISCRETE
  data: noise_state input; filtered_state output; noise_wrench input; filtered_wrench output
function [filtered_state,filtered_wrench] = fcn(noise_state, noise_wrench)
filter_rate = 0.2;
wrench_filter_rate = 0.5;

%% Initialize
persistent quat;
persistent w;
persistent x;
persistent v;
persistent a;
persistent wrench;

if isempty(quat)
    quat = [noise_state(1); noise_state(2); noise_state(3); noise_state(4)];
    w = [noise_state(5); noise_state(6); noise_state(7)];
    x = [noise_state(8); noise_state(9); noise_state(10)];
    v = [noise_state(11); noise_state(12); noise_state(13)];
    a = [noise_state(14); noise_state(15); noise_state(16)];
    wrench = [noise_wrench(1); noise_wrench(2); noise_wrench(3); noise_wrench(4); noise_wrench(5); noise_wrench(6);
              noise_wrench(7); noise_wrench(8); noise_wrench(9); noise_wrench(10); noise_wrench(11); noise_wrench(12)];
end

%% unpack noisy signal
quat_n = [noise_state(1); noise_state(2); noise_state(3); noise_state(4)];
w_n = [noise_state(5); noise_state(6); noise_state(7)];
x_n = [noise_state(8); noise_state(9); noise_state(10)];
v_n = [noise_state(11); noise_state(12); noise_state(13)];
a_n = [noise_state(14); noise_state(15); noise_state(16)];

wrench_n = [noise_wrench(1); noise_wrench(2); noise_wrench(3); noise_wrench(4); noise_wrench(5); noise_wrench(6);
            noise_wrench(7); noise_wrench(8); noise_wrench(9); noise_wrench(10); noise_wrench(11); noise_wrench(12)];

%% filter
quat = filter_rate * quat_n + (1 - filter_rate) * quat;
w = filter_rate * w_n + (1 - filter_rate) * w;
x = filter_rate * x_n + (1 - filter_rate) * x;
v = filter_rate * v_n + (1 - filter_rate) * v;
a = filter_rate * a_n + (1 - filter_rate) * a;
wrench = wrench_filter_rate * wrench_n + (1 - wrench_filter_rate) * wrench;

%% output
filtered_state = [quat; w; x; v; a];
filtered_wrench = wrench;

== matlab function UR5/Controller ==
  settings: updateMethod=DISCRETE  sampleTime=0.0005
  data: ref input; tau_1 output; tau_2 output; Rotation_matrix output; rp input; state input; wrench input; t input; aa output; b output; c output; dbg output; dbg1 output; dbg2 output; dbg3 output; dbg4 output; dbg5 output; dbg6 output; dbg7 output; dbg8 output
function [tau_1,tau_2,Rotation_matrix,aa, b, c, dbg, dbg1, dbg2, dbg3, dbg4, dbg5, dbg6, dbg7, dbg8] = fcn(ref, rp, state, wrench, t)
%% gains
% robot number
N = 2;

% ICL gain
N_o = 150;
eason_integral = 2;%3;
ICL_switcher = true;
k_cl_m = 56000;%18000
k_cl_rp = 63000;
k_cl_I = 25000;
k_cl_Ixx = 23000;
k_cl_Iyy = 42000;
k_cl_Izz = 34000;
k_cl_ri_1 = 67000;%23000
k_cl_ri_2 = 43000;
if N == 1
    k_cl = [k_cl_m k_cl_rp*ones(1,3) k_cl_Ixx k_cl_I k_cl_I k_cl_Iyy k_cl_I k_cl_Izz k_cl_ri_1*ones(1,3)];
else
    k_cl = [k_cl_m k_cl_rp*ones(1,3) k_cl_Ixx k_cl_I k_cl_I k_cl_Iyy k_cl_I k_cl_Izz k_cl_ri_1*ones(1,3) k_cl_ri_2*ones(1,3)];
end
k_cl_gain = diag(k_cl);

% gamma o
g_m = 0.0003;%0.0005
g_rp = 0.0003;%0.02
g_I = 0.001;
g_Ixx = 0.001;
g_Iyy = 0.001;
g_Izz = 0.001;
g_ri_1 = 0.0005;%0.01
g_ri_2 = 0.0005;
if N == 1
    gg = [g_m g_rp*ones(1,3) g_Ixx g_I g_I g_Iyy g_I g_Izz g_ri_1*ones(1,3)];
else
    gg = [g_m g_rp*ones(1,3) g_Ixx g_I g_I g_Iyy g_I g_Izz g_ri_1*ones(1,3) g_ri_2*ones(1,3)];
end
g_o = diag(gg);

% Kd matrix
Kdl = 0.3; %0.3
kdz = 6;
Kdr = 1.2; %0.8
Kdd = [Kdl*ones(1,2) kdz Kdr*ones(1,3)];
Kd = diag(Kdd);

% sliding parameter
lambda = 3;

% deadband in which to stop adaptation
deadband = 0.0;

% Leader switch
leader_switch = 5;
add_on = zeros(6, 2);

% noise mode
noise = false;

%% function definition
function output = vee(matrix)
    output = [matrix(3, 2); matrix(1, 3); matrix(2, 1)];
end

function output = Pa(matrix)
    output = 0.5 * (matrix - matrix.');
end

function output = skew(v)
   output =  [    0 -v(3)   v(2)
               v(3)     0  -v(1)
              -v(2)  v(1)      0];
end

function output = L(v)
    output = [v(1)  v(2)  v(3)     0     0     0
                 0  v(1)     0  v(2)  v(3)     0
                 0     0  v(1)     0  v(2)  v(3)];
end
%% initialize
persistent v_last;
persistent w_last;
persistent index;
persistent mat_matrix;
persistent theta_o_hat;
persistent theta_o;
persistent Rd;
persistent xd;
persistent ICL_update;
persistent t_last;
persistent eason_ptr;
persistent condition;

if isempty(index)
        % ground truth
        mass = 2;
        center_of_mass = rp;
        I = [0.0133333, 0, 0;
              0, 0.0483333, 0;
              0, 0, 0.0483333];
        I_p = I + mass * ((rp * rp.') * diag(ones(1,3)) - rp.' * rp);
        inertia_matrix = [I_p(1) I_p(2) I_p(3) I_p(5) I_p(6) I_p(9)];

        r1 = [-0.25 0 0] - rp;
        r2 = [0.25 0 0] - rp;
        r = [r1, r2];
        if N == 1
            theta_o = [mass mass*center_of_mass inertia_matrix r1].';
        else
            theta_o = [mass mass*center_of_mass inertia_matrix r].';
        end
        
        % initial guess
        theta_o_hat = zeros(10 + 3 * N, 1);
        theta_o_hat = theta_o;
        % mass
        theta_o_hat(1) = 0;
        % COG
        theta_o_hat(2) = 0;
        theta_o_hat(3) = 0;
        theta_o_hat(4) = 0;
        % Inertia
        theta_o_hat(5) = 0.0;
        theta_o_hat(6) = 0.0;
        theta_o_hat(7) = 0.0;
        theta_o_hat(8) = 0.0;
        theta_o_hat(9) = 0.0;
        theta_o_hat(10) = 0.0;
        % 1st grasp point
        theta_o_hat(11) = 0;
        theta_o_hat(12) = 0;
        theta_o_hat(13) = 0;
        % 2nd grasp point
        if N == 2
            theta_o_hat(14) = 0;
            theta_o_hat(15) = 0;
            theta_o_hat(16) = 0;
        end
        
        % without ICL first time
        ICL_update = false;

        Rd = [1  0  0;
              0  1  0;
              0  0  1];

        xd = [0.7250; 0.1092; 0.42] + rp.';
        index = 1;
        v_last = zeros(3, 1);
        w_last = zeros(3, eason_integral);
        mat_matrix = zeros(size(theta_o_hat, 1), N_o);
        t_last = 0;
        eason_ptr = 1;
        condition = 1;
end

mat_sum = zeros(size(theta_o_hat, 1), 1);
debug_msg = zeros(6, 1);
dt = t - t_last;
G = [0; 0; -9.80665];

%% unpack ref
vd = [ref(1); ref(2); ref(3)];
ad = [ref(4); ref(5); ref(6)];
wd = [ref(7); ref(8); ref(9)];
ald = [ref(10); ref(11); ref(12)];

%% unpack state
quat = [state(1) state(2) state(3) state(4)];
R = quat2rotm(quat);
w = [state(5); state(6); state(7)];
x = [state(8); state(9); state(10)];
v = [state(11); state(12); state(13)];
a = [state(14); state(15); state(16)];

%% Noise
if noise == true
    R = rotx(wgn(1, 1, -1)) * roty(wgn(1, 1, -1)) * rotz(wgn(1, 1, -1)) * R;
    w = w + wgn(3, 1, -35);
    x = x + wgn(3, 1, -40);
    v = v + wgn(3, 1, -20);
    a = a + wgn(3, 1, -1) * pi / 180;
end

%% Wrench frame convert
wrench_rotation = [         R, zeros(3,3);
                   zeros(3,3),          R];
wrench1_b = [wrench(1); wrench(2); wrench(3); wrench(4); wrench(5); wrench(6)];
wrench_1 = wrench_rotation * wrench1_b;
force_1 = [wrench_1(1); wrench_1(2); wrench_1(3)];
if N == 2
    wrench2_b = [wrench(7); wrench(8); wrench(9); wrench(10); wrench(11); wrench(12)];
    wrench_2 = wrench_rotation * wrench2_b;
    force_2 = [wrench_2(1); wrench_2(2); wrench_2(3)];
end

%% compute error signals
Re = Rd.' * R;
we = w - wd;

%% compute composite error s
sigma = we + lambda * Rd * vee(Pa(Re));
v_t = v - vd;
x_t = x - xd;
s = [v_t + lambda * x_t;
                  sigma];

%% regression matrix
alpha_r = ald - lambda * skew(wd) * Rd * vee(Pa(Re)) - lambda * Rd * vee(Pa(skew(Rd.' * we) * Re));
w_r = wd - lambda * Rd * vee(Pa(Re));
a_r = ad - lambda * v_t;
v_r = vd - lambda * x_t;

Y_l = [a_r - G, -skew(alpha_r) * R - skew(w) * skew(w_r) * R, zeros(3,6+3*N)];
if N == 1
    Y_r = [zeros(3,1), skew(a_r - G) * R + skew(w) * skew(v_r) * R - skew(w_r) * skew(v) * R, R * L(R.' * alpha_r) + skew(w) * R * L(R.' * w_r), skew(force_1)*R];
else
    Y_r = [zeros(3,1), skew(a_r - G) * R + skew(w) * skew(v_r) * R - skew(w_r) * skew(v) * R, R * L(R.' * alpha_r) + skew(w) * R * L(R.' * w_r), skew(force_1)*R, skew(force_2)*R];
end
Y_o = [Y_l;
       Y_r];
   
%% ICL
if ICL_update && ICL_switcher
    y_l = [(a - G) * eason_integral * dt, -skew(w - w_last(:,eason_ptr)) * R - (skew(w) * skew(w) * R) * eason_integral * dt, zeros(3,6 + 3 * N)];
    if N == 1
        y_r = [zeros(3,1), skew(a - G) * R * eason_integral * dt, R * L(R.' * (w - w_last(:,eason_ptr))) + (skew(w) * R * L(R.' * w)) * eason_integral * dt, skew(force_1) * R * eason_integral * dt];
    else
        y_r = [zeros(3,1), skew(a - G) * R * eason_integral * dt, R * L(R.' * (w - w_last(:,eason_ptr))) + (skew(w) * R * L(R.' * w)) * eason_integral * dt, skew(force_1) * R * eason_integral * dt, skew(force_2) * R * eason_integral * dt];
    end

    y_o_cl_integral = [y_l;
                       y_r];

    if index > N_o
        index = 1;
    end

    if N == 1
        true_tau_integral = wrench_1 * eason_integral * dt;
    else
        true_tau_integral = (wrench_1 + wrench_2) * eason_integral * dt;
    end
    
    y_o_cl_integral_a_hat = y_o_cl_integral * theta_o_hat;
    mat_now = y_o_cl_integral.' * (y_o_cl_integral_a_hat - true_tau_integral);
    
    debug_msg = y_o_cl_integral * theta_o - true_tau_integral;

    
    mat_matrix(:, index) = mat_now;

    mat_sum = sum(mat_matrix, 2);

    index = index + 1;

    v_last = v;
    w_last(:,eason_ptr) = w;
    if eason_ptr >= eason_integral
        eason_ptr = 1;
    else
        eason_ptr = eason_ptr + 1;
    end
end

t_last = t;

theta_o_hat_dot = zeros(10 + 3 * N, 1);
if ICL_update && ICL_switcher
    theta_o_hat_dot = -g_o * Y_o.' * s - k_cl_gain * g_o * mat_sum;
else
    theta_o_hat_dot = -g_o * Y_o.' * s;
end

% decide whether update or not
if norm(s) < deadband
    ICL_update = false;
else
    ICL_update = true;
end

%% desired signal calculate
Rd = expm(dt * skew(wd)) * Rd; % Matrix Exponential
xd = xd + vd * dt + 0.5 * ad * dt * dt;

%% update law
theta_o_hat = theta_o_hat + theta_o_hat_dot * dt;
% theta_o_hat(5:10) = max(theta_o_hat(5:10), 0);

%% controller
tau = -Kd * s;
tau = min(max(tau, -20),40);

%% leader switch
if mod(t, leader_switch) == 0
    condition = mod((condition + 1), N); % condition = 0 or 1
end
if condition == 0
    add_on = [Y_o * theta_o_hat, zeros(6, 1)];
else
    add_on = [zeros(6, 1), Y_o * theta_o_hat];
end

%% output
tau_1 = tau + add_on(:, 1);
tau_2 = tau + add_on(:, 2);
% tau_1 = tau;
% tau_2 = tau;
Rotation_matrix = R;
aa = x_t;
b = theta_o - theta_o_hat;
c = norm(s);
dbg = x;
dbg1 = xd;
dbg2 = v;
dbg3 = vd;
dbg4 = w;
dbg5 = wd;
dbg6 = norm(s);
dbg7 = 3 - trace(Re);
dbg8 = theta_o_hat;
end

== matlab function UR5/TH Magic/Arm 1 Magic/Transformation ==
  settings: updateMethod=DISCRETE  sampleTime=0.0005
  data: translation input; RPY input; T output
function T = fcn(translation, RPY)
    persistent R;
    persistent R_i;
    if isempty(R)
%         R = diag(ones(1,3));
         R = [1     0     0;
              0    -1     0;
              0     0    -1];
         R_i = R;
    end

R = rotx(RPY(1)) * roty(RPY(2)) * rotz(RPY(3)) * R; % *180/pi
T = [R translation;
     zeros(1,3)  1
    ];

== matlab function UR5/TH Magic/Arm 2 Magic/Transformation ==
  settings: updateMethod=DISCRETE  sampleTime=0.0005
  data: translation input; RPY input; T output
function T = fcn(translation, RPY)
    persistent R;
    persistent R_i;
    if isempty(R)
%         R = diag(ones(1,3));
         R = [1     0     0;
              0    -1     0;
              0     0    -1];
         R_i = R;
    end

R = rotx(RPY(1)) * roty(RPY(2)) * rotz(RPY(3)) * R; % *180/pi
T = [R translation;
     zeros(1,3)  1
    ];

== matlab function UR5/TH Magic/Arm 1 Magic/Wrench Converter ==
  settings: updateMethod=DISCRETE  sampleTime=0.0001
  data: w_b input; wrench_world output; R input
function wrench_world = fcn(w_b, R)
wrench_rotation = [         R, zeros(3,3);
                   zeros(3,3),          R];
wrench_world = wrench_rotation * w_b;

== matlab function UR5/TH Magic/Arm 2 Magic/Wrench Converter ==
  settings: updateMethod=DISCRETE  sampleTime=0.0001
  data: w_b input; wrench_world output; R input
function wrench_world = fcn(w_b, R)
wrench_rotation = [         R, zeros(3,3);
                   zeros(3,3),          R];
wrench_world = wrench_rotation * w_b;

== matlab function UR5/TH Magic/Arm 1 Magic/Low Pass Filter ==
  data: u input; y output
function y = fcn(u)
rate = 0.8;
persistent wrench_last;
if isempty(wrench_last)
    wrench_last = zeros(6,1);
end
y = rate * u + (1 - rate) * wrench_last;
wrench_last = y;

== matlab function UR5/TH Magic/Arm 2 Magic/Low Pass Filter ==
  data: u input; y output
function y = fcn(u)
rate = 0.8;
persistent wrench_last;
if isempty(wrench_last)
    wrench_last = zeros(6,1);
end
y = rate * u + (1 - rate) * wrench_last;
wrench_last = y;

== matlab function UR5/Low Pass Filter ==
  settings: updateMethod=DISCRETE  sampleTime=0.001
  data: u input; y output
function y = fcn(u)
rate = 0.8;
persistent wrench_last;
if isempty(wrench_last)
    wrench_last = zeros(12,1);
end
y = rate * u + (1 - rate) * wrench_last;
wrench_last = y;
